simulink library "VehicleSimulation"  (R2014a)
settings: Solver=ode45  SolverMode=SingleTasking  StartTime=0.0  StopTime=10.0  RelTol=1e-3
undefined symbols (not defined in the file): bs, eff, fs, gpsins, gr, Js, kM, ljt, lma, param, rjt, rma, sglu, sr
libraries: simulink x2, VehicleSimulation x1
(part 1 of 2)
settings Model: Creator=Administrator  LastModifiedBy=cbeal

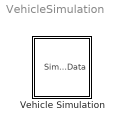
== system VehicleSimulation ==
  Vehicle Simulation : Subsystem  StopFcn=|  mask{InitPosE=9362.6, InitPosN=-418.6, InitYawAngle=-81.2, CruiseEnableTime=1, AutoSteerEnable=on, FaultEnable=off, HWHALEnable=off, TwoWheelEnable=on, DiffDriveEnable=off}
      | DataDescription = datadesc;                          
      | DataDescriptionSimulation=datadescSimulation;        
      |                                                      
      | %DataDescriptionUser = %datadescDriftController      
      |                                                      
      | %DataDescriptionUser = %datadescDriftSpeedController;
      |                                                      
      | DataDescriptionUser = datadescDriftkeeping;          
      |                                                      
      | %DataDescriptionUser = %datadescDriftControllerSDSC; 
      |                                                      
      | names;
      mask prompts: InitPosE "Initial East Position"; InitPosN "Initial North Position"; InitYawAngle "Initial Yaw Angle (deg)"; CruiseEnableTime "Cruise Control Enable Time (s)"; AutoSteerEnable "Enable Auto Steer"; FaultEnable "Enable Faults"; HWHALEnable "Enable HAL HW"; TwoWheelEnable "Use Two Wheel Model"; DiffDriveEnable "Use Differential Drive"
      mask help: This block provides a simulated hardware model.
      mask init:
      | InitModel;
      | p1_params;
      | ssest_params;
      | sim_params;
      | 
      | % TwoWheelSwitch_DriftControl = [gcs '/User Controllers' '/Drift and Speed Controller' '/Drift Controller Subsystem' '/Use Two Wheel Model'];
      | % TwoWheelSwitch_DriftControl = [gcs '/User Controllers' '/Simplified Drift Control' '/Drift Controller Subsystem' '/Use Two Wheel Model'];
      | % TwoWheelSwitch_DriftControl = [gcs '/User Controllers' '/Drift Control Block' '/Drift Controller Subsystem' '/Use Two Wheel Model'];
      | TwoWheelSwitch_DriftControl = [gcs '/User Controllers' '/Driftkeeping' '/Driftkeeping Subsystem' '/Use Two Wheel Model'];
      | TwoWheelSwitch_Sim = [gcs '/Vehicle Simulation' '/Vehicle Model' '/Use Two Wheel Model'];
      | DifferentialSwitch_Sim = [gcs '/Vehicle Simulation' '/Vehicle Model' '/Use Differential Drive'];
      | hwhal = [gcs '/Vehicle Simulation' '/Driver' '/Handwheel System' '/Enable HALHW'];
      | 
      | % default is turn off hwhal, two wheel model
      | set_param(hwhal, 'value', '0');
      | set_param(TwoWheelSwitch_DriftControl, 'value', '0');
      | set_param(TwoWheelSwitch_Sim, 'value', '0');
      | set_param(DifferentialSwitch_Sim, 'value', '0');
      | 
      | if (HWHALEnable == 1)
      |     set_param(hwhal, 'value', '1');
      | end
      | 
      | if (TwoWheelEnable == 1)
      |     set_param(TwoWheelSwitch_DriftControl, 'value', '1');
      |     set_param(TwoWheelSwitch_Sim, 'value', '1');
      | end
      | 
      | if (DiffDriveEnable == 1)
      |     set_param(DifferentialSwitch_Sim, 'value', '1');
      | end
      mask Display: disp('Sim');

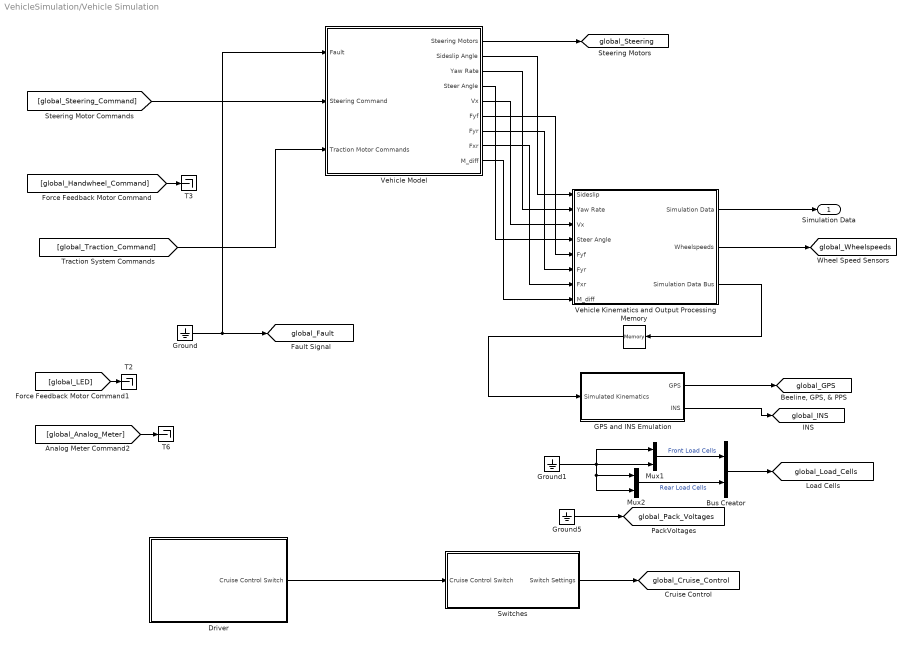
== system VehicleSimulation/Vehicle Simulation ==
  Bus Creator : BusCreator  Inputs=2
  Driver : Subsystem
  GPS and INS Emulation : Subsystem
  Ground : Ground
  Ground1 : Ground
  Ground5 : Ground
  Memory : Memory
  Mux1 : Mux  Inputs=2
  Mux2 : Mux  Inputs=2
  Switches : Subsystem
  T2 : Terminator
  T3 : Terminator
  T6 : Terminator
  Vehicle Kinematics and Output Processing : Subsystem
  Vehicle Model : Subsystem
  Simulation Data : Outport
  tag scope: global_Cruise_Control=global, global_Fault=global, global_GPS=global, global_INS=global, global_Load_Cells=global, global_Pack_Voltages=global, global_Steering=global, global_Wheelspeeds=global
  wires:
  Memory/1 -> GPS and INS Emulation/1(Simulated Kinematics)
  Vehicle Kinematics and Output Processing/3(Simulation Data Bus) -> Memory/1
  Vehicle Model/9(M_diff) -> Vehicle Kinematics and Output Processing/8(M_diff)
  Ground1/1 -> Mux2/2, Mux2/1, Mux1/2, Mux1/1
  GPS and INS Emulation/2(INS) -> [global_INS]
  GPS and INS Emulation/1(GPS) -> [global_GPS]
  Mux2/1 -> Bus Creator/2  "Rear Load Cells"
  Mux1/1 -> Bus Creator/1  "Front Load Cells"
  Driver/1(Cruise Control Switch) -> Switches/1(Cruise Control Switch)
  Vehicle Model/2(Sideslip Angle) -> Vehicle Kinematics and Output Processing/1(Sideslip)
  Vehicle Model/3(Yaw Rate) -> Vehicle Kinematics and Output Processing/2(Yaw Rate)
  Vehicle Model/1(Steering Motors) -> [global_Steering]
  Ground/1 -> Vehicle Model/1(Fault), [global_Fault]
  [global_Handwheel_Command] -> T3/1
  [global_LED] -> T2/1
  [global_Analog_Meter] -> T6/1
  Bus Creator/1 -> [global_Load_Cells]
  Ground5/1 -> [global_Pack_Voltages]
  Vehicle Kinematics and Output Processing/1(Simulation Data) -> Simulation Data/1
  Switches/1(Switch Settings) -> [global_Cruise_Control]
  [global_Steering_Command] -> Vehicle Model/2(Steering Command)
  Vehicle Model/4(Steer Angle) -> Vehicle Kinematics and Output Processing/4(Steer Angle)
  [global_Traction_Command] -> Vehicle Model/3(Traction Motor Commands)
  Vehicle Model/5(Vx) -> Vehicle Kinematics and Output Processing/3(Vx)
  Vehicle Model/6(Fyf) -> Vehicle Kinematics and Output Processing/5(Fyf)
  Vehicle Model/7(Fyr) -> Vehicle Kinematics and Output Processing/6(Fyr)
  Vehicle Model/8(Fxr) -> Vehicle Kinematics and Output Processing/7(Fxr)
  Vehicle Kinematics and Output Processing/2(Wheelspeeds) -> [global_Wheelspeeds]

== system VehicleSimulation/Vehicle Simulation/Driver ==
  Ground6 : Ground
  Handwheel System : Subsystem
  Pedal Voltage : Constant  Value=1.95
  Step : Step  Time=CruiseEnableTime  SampleTime=0
  Step1 : Step  Time=CruiseEnableTime+0.1  After=-1  SampleTime=0
  Sum : Sum  Inputs=+|+
  Cruise Control Switch : Outport
  tag scope: global_Go_Pedal=global, global_Handwheel=global, global_Prerecorded_Steering_Command=global
  wires:
  Step1/1 -> Sum/2
  Step/1 -> Sum/1
  Sum/1 -> Cruise Control Switch/1
  Ground6/1 -> [global_Prerecorded_Steering_Command]
  Pedal Voltage/1 -> [global_Go_Pedal]
  Handwheel System/1(Handwheel Signals) -> [global_Handwheel]

== system VehicleSimulation/Vehicle Simulation/GPS and INS Emulation ==
  Simulated Kinematics : Inport
  Bus Selector : BusSelector  OutputSignals=Yaw Rate,Heading,ax,ay,Vx,Vy,Pos E,Pos N
  Emulated INS : Subsystem
  GPS Emulation : Subsystem
  Radians to Degrees : Gain  Gain=180/pi
  Shift to Sensor/GPS Positions : Subsystem
  GPS : Outport
  INS : Outport  Port=2
  wires:
  Emulated INS/1(INS) -> INS/1
  GPS Emulation/1(Emulated GPS) -> GPS/1
  Shift to Sensor/GPS Positions/1(axINS) -> Emulated INS/2(axINS)
  Bus Selector/2 -> Radians to Degrees/1  "<Heading>"
  Radians to Degrees/1 -> GPS Emulation/1(Heading Angle)
  Bus Selector/4 -> Emulated INS/3(ay)  "<ay>"
  Bus Selector/8 -> GPS Emulation/5(Pos N)  "<Pos N>"
  Shift to Sensor/GPS Positions/2(VyGPS) -> GPS Emulation/3(VyGPS)
  Bus Selector/7 -> GPS Emulation/4(Pos E)  "<Pos E>"
  Bus Selector/6 -> Shift to Sensor/GPS Positions/3(Vy)  "<Vy>"
  Bus Selector/5 -> GPS Emulation/2(Vx)  "<Vx>"
  Bus Selector/3 -> Shift to Sensor/GPS Positions/2(ax)  "<ax>"
  Bus Selector/1 -> Emulated INS/1(Yaw Rate), Shift to Sensor/GPS Positions/1(Yaw Rate)  "<Yaw Rate>"
  Simulated Kinematics/1 -> Bus Selector/1

== system VehicleSimulation/Vehicle Simulation/Switches ==
  Cruise Control Switch : Inport
  Auto-Steer Switch : Constant  Value=AutoSteerEnable
  Brakes Disabled : Constant  Value=0
  Fault Switch : Constant  Value=FaultEnable
  Mux : Mux
  Switch Settings : Outport
  wires:
  Brakes Disabled/1 -> Mux/4  "Brake Pedal Signal"
  Auto-Steer Switch/1 -> Mux/2  "Auto-Steer Switch"
  Cruise Control Switch/1 -> Mux/3  "Cruise Control Switch"
  Fault Switch/1 -> Mux/1  "Fault Switch"
  Mux/1 -> Switch Settings/1

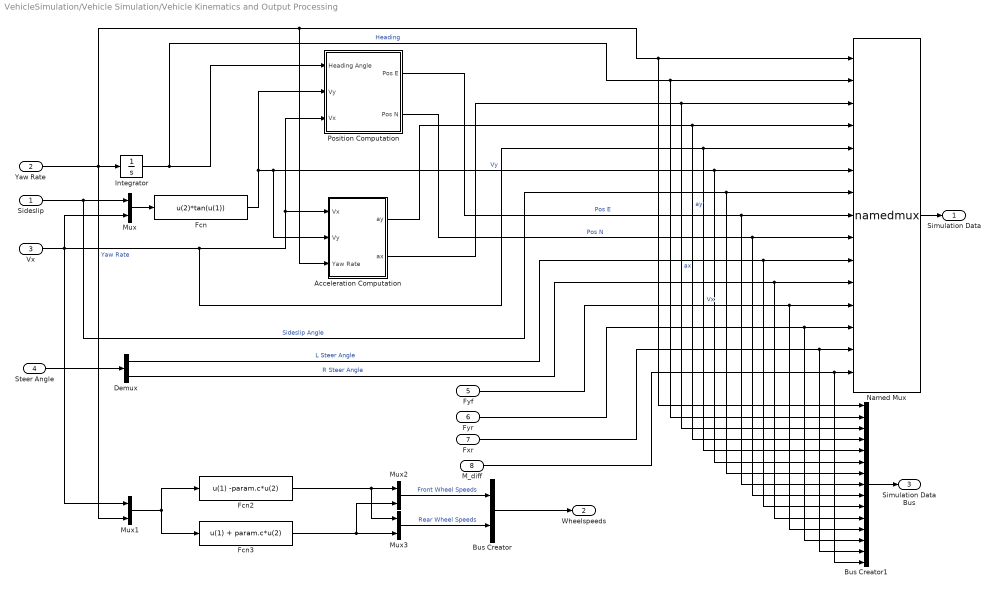
== system VehicleSimulation/Vehicle Simulation/Vehicle Kinematics and Output Processing ==
  Sideslip : Inport
  Yaw Rate : Inport  Port=2
  Vx : Inport  Port=3
  Steer Angle : Inport  Port=4
  Fyf : Inport  Port=5
  Fyr : Inport  Port=6
  Fxr : Inport  Port=7
  M_diff : Inport  Port=8
  Acceleration Computation : Subsystem
  Bus Creator : BusCreator  Inputs=2
  Bus Creator1 : BusCreator  Inputs=15
  Demux : Demux  Outputs=2
  Fcn : Fcn  Expr=u(2)*tan(u(1))
  Fcn2 : Fcn  Expr=u(1) -param.c*u(2)
  Fcn3 : Fcn  Expr=u(1) + param.c*u(2)
  Integrator : Integrator  InitialCondition=InitYawAngle*(pi/180)
  Mux{,1..3} (4 alike) : Mux  Inputs=2
  Named Mux : S-Function  FunctionName=namedmux  Parameters=inputcount,inputsizes  EnableBusSupport=off  mask{fname=datadescSimulation}
      mask prompts: fname "Data description function name"
      mask help:
      | Combines input signals into a single output vector, according to a structure that provides the names and sizes of each signal.
      |
      | The parameter below should be set to the name of a function which returns a 1xN structure array, where N is the number of input signals.  The structure should contain fields "size" which specifies the width of the input signal, and "name" which specifies its name.
      mask init:
      | desc=eval(fname);
      | %if(class(desc)~='cell')
      | %	error('Incorrect description');
      | %end
      | inputcount=length(desc);
      | if((inputcount<1)|(inputcount>50))
      | 	error('Inappropriate number of inputs.');
      | end
      | 
      | inputsizes=[desc.size];
      | 
      | x=min(inputcount*ones(1,50),1:50);
      mask Display:
      | port_label('input',x(1),desc(x(1)).name);
      | port_label('input',x(2),desc(x(2)).name);
      | port_label('input',x(3),desc(x(3)).name);
      | port_label('input',x(4),desc(x(4)).name);
      | port_label('input',x(5),desc(x(5)).name);
      | port_label('input',x(6),desc(x(6)).name);
      | port_label('input',x(7),desc(x(7)).name);
      | port_label('input',x(8),desc(x(8)).name);
      | port_label('input',x(9),desc(x(9)).name);
      | port_label('input',x(10),desc(x(10)).name);
      | port_label('input',x(11),desc(x(11)).name);
      | port_label('input',x(12),desc(x(12)).name);
      | port_label('input',x(13),desc(x(13)).name);
      | port_label('input',x(14),desc(x(14)).name);
      | port_label('input',x(15),desc(x(15)).name);
      | port_label('input',x(16),desc(x(16)).name);
      | port_label('input',x(17),desc(x(17)).name);
      | port_label('input',x(18),desc(x(18)).name);
      | port_label('input',x(19),desc(x(19)).name);
      | port_label('input',x(20),desc(x(20)).name);
      | port_label('input',x(21),desc(x(21)).name);
      | port_label('input',x(22),desc(x(22)).name);
      | port_label('input',x(23),desc(x(23)).name);
      | port_label('input',x(24),desc(x(24)).name);
      | port_label('input',x(25),desc(x(25)).name);
      | port_label('input',x(26),desc(x(26)).name);
      | port_label('input',x(27),desc(x(27)).name);
      | port_label('input',x(28),desc(x(28)).name);
      | port_label('input',x(29),desc(x(29)).name);
      | port_label('input',x(30),desc(x(30)).name);
  Position Computation : Subsystem
  Simulation Data : Outport
  Wheelspeeds : Outport  Port=2
  Simulation Data Bus : Outport  Port=3
  wires:
  M_diff/1 -> Bus Creator1/15, Named Mux/15
  Integrator/1 -> Position Computation/1(Heading Angle), Named Mux/2, Bus Creator1/2  "Heading"
  Fcn/1 -> Position Computation/2(Vy), Acceleration Computation/2(Vy), Named Mux/6, Bus Creator1/6  "Vy"
  Sideslip/1 -> Mux/1, Bus Creator1/7, Named Mux/7  "Sideslip Angle"
  Mux/1 -> Fcn/1
  Vx/1 -> Mux/2, Position Computation/3(Vx), Acceleration Computation/1(Vx), Named Mux/5, Bus Creator1/5, Mux1/1  "Vx"
  Yaw Rate/1 -> Acceleration Computation/3(Yaw Rate), Named Mux/1, Bus Creator1/1, Integrator/1, Mux1/2  "Yaw Rate"
  Position Computation/1(Pos E) -> Named Mux/8, Bus Creator1/8  "Pos E"
  Position Computation/2(Pos N) -> Named Mux/9, Bus Creator1/9  "Pos N"
  Named Mux/1 -> Simulation Data/1
  Steer Angle/1 -> Demux/1
  Demux/1 -> Named Mux/10, Bus Creator1/10  "L Steer Angle"
  Demux/2 -> Named Mux/11, Bus Creator1/11  "R Steer Angle"
  Acceleration Computation/1(ay) -> Named Mux/4, Bus Creator1/4  "ay"
  Acceleration Computation/2(ax) -> Named Mux/3, Bus Creator1/3  "ax"
  Fyf/1 -> Named Mux/12, Bus Creator1/12
  Fyr/1 -> Named Mux/13, Bus Creator1/13
  Fxr/1 -> Named Mux/14, Bus Creator1/14
  Mux1/1 -> Fcn2/1, Fcn3/1
  Fcn2/1 -> Mux2/1, Mux3/1
  Fcn3/1 -> Mux3/2, Mux2/2
  Mux2/1 -> Bus Creator/1  "Front Wheel Speeds"
  Mux3/1 -> Bus Creator/2  "Rear Wheel Speeds"
  Bus Creator/1 -> Wheelspeeds/1
  Bus Creator1/1 -> Simulation Data Bus/1

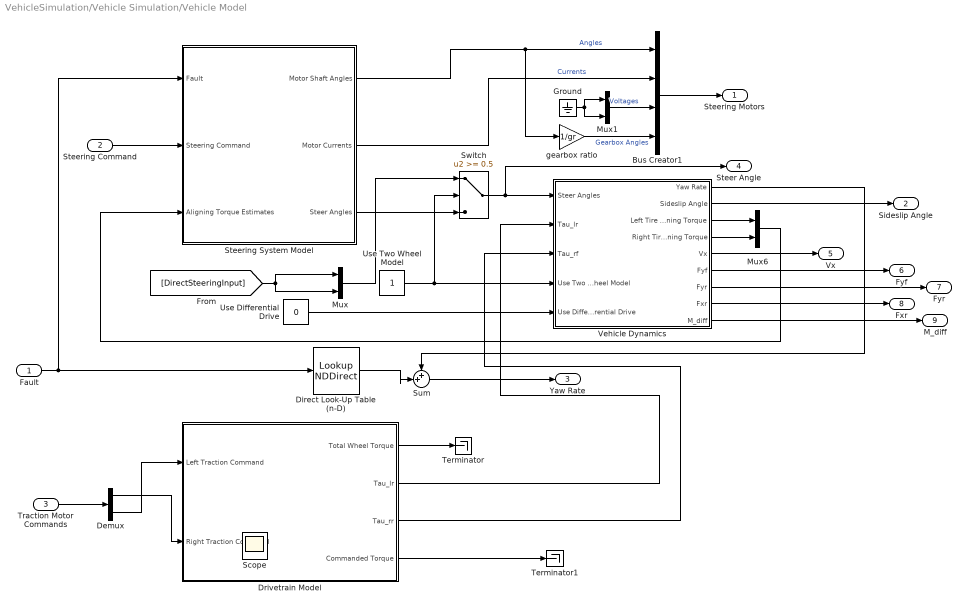
== system VehicleSimulation/Vehicle Simulation/Vehicle Model ==
  Fault : Inport
  Steering Command : Inport  Port=2
  Traction Motor Commands : Inport  Port=3
  Bus Creator1 : BusCreator
  Demux : Demux  Outputs=2
  Direct Look-Up Table (n-D) : LookupNDDirect  NumberOfTableDimensions=1  Table=[0 0 0 0 0 .01]
  Drivetrain Model : Subsystem
  Ground : Ground
  Mux : Mux  Inputs=2
  Mux1 : Mux  Inputs=2
  Mux6 : Mux  Inputs=2
  Scope : Scope
  Steering System Model : Subsystem
  Sum : Sum  Inputs=++|
  Switch : Switch  Threshold=0.5
  Terminator : Terminator
  Terminator1 : Terminator
  Use Differential Drive : Constant  Value=0
  Use Two Wheel Model : Constant
  Vehicle Dynamics : Subsystem
  gearbox ratio : Gain  Gain=1/gr  SaturateOnIntegerOverflow=on  OutDataTypeStr=Inherit: Same as input  ParamDataTypeStr=Inherit: Same as input
  Steering Motors : Outport
  Sideslip Angle : Outport  Port=2
  Yaw Rate : Outport  Port=3
  Steer Angle : Outport  Port=4
  Vx : Outport  Port=5
  Fyf : Outport  Port=6
  Fyr : Outport  Port=7
  Fxr : Outport  Port=8
  M_diff : Outport  Port=9
  wires:
  Drivetrain Model/3(Tau_rr) -> Vehicle Dynamics/3(Tau_rf)
  Drivetrain Model/2(Tau_lr) -> Vehicle Dynamics/2(Tau_lr)
  Vehicle Dynamics/9(M_diff) -> M_diff/1
  Traction Motor Commands/1 -> Demux/1
  Mux/1 -> Switch/1
  Steering System Model/3(Steer Angles) -> Switch/3
  Switch/1 -> Steer Angle/1, Vehicle Dynamics/1(Steer Angles)
  [DirectSteeringInput] -> Mux/2, Mux/1
  Vehicle Dynamics/2(Sideslip Angle) -> Sideslip Angle/1
  Sum/1 -> Yaw Rate/1
  Vehicle Dynamics/4(Right Tire Aligning Torque) -> Mux6/2
  Vehicle Dynamics/3(Left Tire Aligning Torque) -> Mux6/1
  Bus Creator1/1 -> Steering Motors/1
  Steering System Model/1(Motor Shaft Angles) -> Bus Creator1/1, gearbox ratio/1  "Angles"
  gearbox ratio/1 -> Bus Creator1/4  "Gearbox Angles"
  Steering System Model/2(Motor Currents) -> Bus Creator1/2  "Currents"
  Mux1/1 -> Bus Creator1/3  "Voltages"
  Direct Look-Up Table (n-D)/1 -> Sum/2
  Vehicle Dynamics/1(Yaw Rate) -> Sum/1
  Fault/1 -> Steering System Model/1(Fault), Direct Look-Up Table (n-D)/1
  Steering Command/1 -> Steering System Model/2(Steering Command)
  Mux6/1 -> Steering System Model/3(Aligning Torque Estimates)
  Vehicle Dynamics/5(Vx) -> Vx/1
  Drivetrain Model/1(Total Wheel Torque) -> Terminator/1
  Drivetrain Model/4(Commanded Torque) -> Terminator1/1
  Vehicle Dynamics/6(Fyf) -> Fyf/1
  Vehicle Dynamics/7(Fyr) -> Fyr/1
  Vehicle Dynamics/8(Fxr) -> Fxr/1
  Ground/1 -> Mux1/1, Mux1/2
  Use Two Wheel Model/1 -> Vehicle Dynamics/4(Use Two Wheel Model), Switch/2
  Use Differential Drive/1 -> Vehicle Dynamics/5(Use Differential Drive)
  Demux/2 -> Drivetrain Model/1(Left Traction Command)
  Demux/1 -> Drivetrain Model/2(Right Traction Command)

== system VehicleSimulation/Vehicle Simulation/Driver/Handwheel System ==
  Bus Creator3 : BusCreator  Inputs=3
  Enable HALHW : Constant  Value=0
  Ground : Ground
  Ground1 : Ground
  HAL-9000 : Subsystem  mask{enabled=on, maneuver=Step, amplitude=10, delay=10, duration=15, startfreq=.7, endfreq=.7}
      mask prompts: enabled "Enable HAL-9000 Automated Steering Maneuver System"; maneuver "Steering manuever"; amplitude "Amplitude (deg)"; delay "Delay (sec)"; duration "Duration (sec)"; startfreq "Initial frequency (Hz)"; endfreq "Final frequency (Hz)"
      mask init:
      | p1_params;
      | SteeringController;
      | 
      | switch(maneuver)
      | 	case 'Step'
      | 		maneuver=1;
      | 	case 'Ramp'
      | 		maneuver=2;
      | 	case 'Chirp'
      | 		maneuver=3;
      | 	case 'Double-step'
      | 		maneuver=4;
      | 	case 'Double chirp'
      | 		maneuver=5;
      | end
      | switch(enabled)
      | 	case 'on'
      | 		enabled=1;
      | 	case 'off'
      | 		enabled=0;
      | end
      mask Callback enabled:
      | if(strcmp(get_param(gcb,'enabled'),'off'))
      | 	set_param(gcb,'MaskEnables',{'on','off','off','off','off','off','off'});
      | else
      | 	set_param(gcb,'MaskEnables',{'on','on','on','on','on','on','on'});
      | end
      mask TypeOptions maneuver: Step | Ramp | Chirp | Double step | Double chirp
      mask Callback maneuver:
      | switch(get_param(gcb,'maneuver'))
      | 	case 'Step'
      | 		set_param(gcb,'MaskVisibilities',{'on','on','on','on','off','off','off'});
      | 	case 'Double step'
      | 		set_param(gcb,'MaskVisibilities',{'on','on','on','on','on','off','off'});
      | 	case 'Ramp'
      | 		set_param(gcb,'MaskVisibilities',{'on','on','on','on','on','off','off'});
      | 	case 'Chirp'
      | 		set_param(gcb,'MaskVisibilities',{'on','on','on','on','on','on','on'});
      | 	case 'Double chirp'
      | 		set_param(gcb,'MaskVisibilities',{'on','on','on','on','on','on','on'});
      | end
  Handwheel Signals : Outport
  wires:
  Enable HALHW/1 -> HAL-9000/1(Trigger)
  HAL-9000/1(Offset) -> Bus Creator3/1  "Primary"
  Ground/1 -> Bus Creator3/2  "First Backup"
  Bus Creator3/1 -> Handwheel Signals/1
  Ground1/1 -> Bus Creator3/3  "Second Backup"

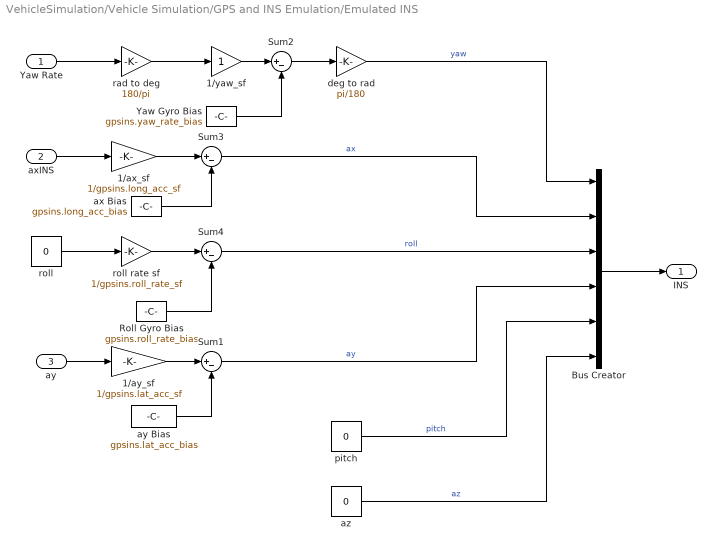
== system VehicleSimulation/Vehicle Simulation/GPS and INS Emulation/Emulated INS ==
  Yaw Rate : Inport
  axINS : Inport  Port=2
  ay : Inport  Port=3
  1/ax_sf : Gain  Gain=1/gpsins.long_acc_sf  SaturateOnIntegerOverflow=on  OutDataTypeStr=Inherit: Same as input  ParamDataTypeStr=Inherit: Same as input
  1/ay_sf : Gain  Gain=1/gpsins.lat_acc_sf  SaturateOnIntegerOverflow=on  OutDataTypeStr=Inherit: Same as input  ParamDataTypeStr=Inherit: Same as input
  1/yaw_sf : Gain
  Bus Creator : BusCreator  Inputs=6
  Roll Gyro Bias : Constant  Value=gpsins.roll_rate_bias
  Sum{1..4} (4 alike) : Sum  Inputs=|+-  SaturateOnIntegerOverflow=on  InputSameDT=on  OutDataTypeStr=Inherit: Same as first input
  Yaw Gyro Bias : Constant  Value=gpsins.yaw_rate_bias
  ax Bias : Constant  Value=gpsins.long_acc_bias
  ay Bias : Constant  Value=gpsins.lat_acc_bias
  az : Constant  Value=0
  deg to rad : Gain  Gain=pi/180
  pitch : Constant  Value=0
  rad to deg : Gain  Gain=180/pi
  roll : Constant  Value=0
  roll rate sf : Gain  Gain=1/gpsins.roll_rate_sf  SaturateOnIntegerOverflow=on  OutDataTypeStr=Inherit: Same as input  ParamDataTypeStr=Inherit: Same as input
  INS : Outport
  wires:
  Bus Creator/1 -> INS/1
  az/1 -> Bus Creator/6  "az"
  pitch/1 -> Bus Creator/5  "pitch"
  Sum4/1 -> Bus Creator/3  "roll"
  Roll Gyro Bias/1 -> Sum4/2
  roll rate sf/1 -> Sum4/1
  roll/1 -> roll rate sf/1
  Sum1/1 -> Bus Creator/4  "ay"
  Sum3/1 -> Bus Creator/2  "ax"
  deg to rad/1 -> Bus Creator/1  "yaw"
  ax Bias/1 -> Sum3/2
  1/ax_sf/1 -> Sum3/1
  axINS/1 -> 1/ax_sf/1
  ay Bias/1 -> Sum1/2
  1/ay_sf/1 -> Sum1/1
  ay/1 -> 1/ay_sf/1
  Sum2/1 -> deg to rad/1
  Yaw Gyro Bias/1 -> Sum2/2
  1/yaw_sf/1 -> Sum2/1
  rad to deg/1 -> 1/yaw_sf/1
  Yaw Rate/1 -> rad to deg/1

== system VehicleSimulation/Vehicle Simulation/GPS and INS Emulation/GPS Emulation ==
  Heading Angle : Inport
  Vx : Inport  Port=2
  VyGPS : Inport  Port=3
  Pos E : Inport  Port=4
  Pos N : Inport  Port=5
  Beeline Emulation : Subsystem
  Bus Creator : BusCreator  Inputs=5
  Clock : Clock
  OEM4 Emulation : Subsystem
  Pulse Generator : DiscretePulseGenerator  PulseType=Time based  Amplitude=4.1  Period=1  PulseWidth=50
  Sum : Sum  Inputs=|++
  UTC Offset : Constant  Value=250000
  Emulated GPS : Outport
  wires:
  OEM4 Emulation/3(OEM4 Other) -> Bus Creator/5  "OEM4 Other"
  OEM4 Emulation/1(OEM4 Position) -> Bus Creator/4  "OEM4 Position"
  Bus Creator/1 -> Emulated GPS/1
  Pulse Generator/1 -> Bus Creator/3  "PPS"
  OEM4 Emulation/2(OEM4 Velocity) -> Bus Creator/2  "OEM4 Velocity"
  Beeline Emulation/1(Beeline) -> Bus Creator/1  "Beeline"
  Pos N/1 -> OEM4 Emulation/5(Pos N)
  Pos E/1 -> OEM4 Emulation/4(Pos E)
  Heading Angle/1 -> Beeline Emulation/1("Heading Angle "), OEM4 Emulation/3(Heading Angle)
  VyGPS/1 -> Beeline Emulation/3(VyGPS), OEM4 Emulation/2(VyGPS)
  Vx/1 -> Beeline Emulation/2(Vx), OEM4 Emulation/1(Vx)
  Sum/1 -> OEM4 Emulation/6(UTC), Beeline Emulation/4(UTC)
  Clock/1 -> Sum/2
  UTC Offset/1 -> Sum/1

== system VehicleSimulation/Vehicle Simulation/GPS and INS Emulation/Shift to Sensor//GPS Positions ==
  Yaw Rate : Inport
  ax : Inport  Port=2
  Vy : Inport  Port=3
  "CG to INS Cube " : Fcn  Expr=u[2] + u[1]^2*gpsins.dist_sensor
  CG to INS Cube 1 : Fcn  Expr=u[2] -u[1]*gpsins.dist_sensor
  INS Cube to GPS Antenna : Fcn  Expr=u[2] + u[1]*gpsins.l_gps_ant
  Mux : Mux  Inputs=2
  Mux1 : Mux  Inputs=2
  Mux2 : Mux  Inputs=2
  axINS : Outport
  VyGPS : Outport  Port=2
  wires:
  "CG to INS Cube "/1 -> axINS/1
  INS Cube to GPS Antenna/1 -> VyGPS/1
  Vy/1 -> Mux1/2
  ax/1 -> Mux/2
  CG to INS Cube 1/1 -> Mux2/2
  Mux2/1 -> INS Cube to GPS Antenna/1
  Mux1/1 -> CG to INS Cube 1/1
  Mux/1 -> "CG to INS Cube "/1
  Yaw Rate/1 -> Mux2/1, Mux/1, Mux1/1

== system VehicleSimulation/Vehicle Simulation/Vehicle Kinematics and Output Processing/Acceleration Computation ==
  Vx : Inport
  Vy : Inport  Port=2
  Yaw Rate : Inport  Port=3
  Derivative : Derivative
  Derivative1 : Derivative
  Fcn1 : Fcn  Expr=u[1] + u[2]*u[3]
  Fcn2 : Fcn  Expr=u[1] - u[2]*u[3]
  Mux : Mux  Inputs=3
  Mux1 : Mux  Inputs=3
  ay : Outport
  ax : Outport  Port=2
  wires:
  Vx/1 -> Mux/3, Derivative/1
  Fcn1/1 -> ay/1
  Mux/1 -> Fcn1/1
  Fcn2/1 -> ax/1
  Mux1/1 -> Fcn2/1
  Derivative1/1 -> Mux/1
  Yaw Rate/1 -> Mux/2, Mux1/2
  Derivative/1 -> Mux1/1
  Vy/1 -> Derivative1/1, Mux1/3

== system VehicleSimulation/Vehicle Simulation/Vehicle Kinematics and Output Processing/Position Computation ==
  Heading Angle : Inport
  Vy : Inport  Port=2
  Vx : Inport  Port=3
  Compute Velocity East : Fcn  Expr=-u(3)*sin(u(1))-u(2)*cos(u(1))
  Computer Velocity North : Fcn  Expr=u(3)*cos(u(1))-u(2)*sin(u(1))
  Integrator : Integrator  InitialCondition=InitPosE
  Integrator1 : Integrator  InitialCondition=InitPosN
  Mux : Mux  Inputs=3
  Pos E : Outport
  Pos N : Outport  Port=2
  wires:
  Integrator1/1 -> Pos N/1
  Integrator/1 -> Pos E/1
  Mux/1 -> Computer Velocity North/1, Compute Velocity East/1
  Vx/1 -> Mux/3
  Vy/1 -> Mux/2
  Heading Angle/1 -> Mux/1
  Compute Velocity East/1 -> Integrator/1
  Computer Velocity North/1 -> Integrator1/1

== system VehicleSimulation/Vehicle Simulation/Vehicle Model/Drivetrain Model ==
  Left Traction Command : Inport
  Right Traction Command : Inport  Port=2
  Drivetrain Model : Subsystem  TreatAsAtomicUnit=on
  Lookup Table : Lookup  InputValues=[0.9,1.7,2.8]  Table=[-70.5,0,190.5]  LookUpMeth=Interpolation-Use End Values
  Lookup Table1 : Lookup  InputValues=[0.9,1.7,2.8]  Table=[-70.5,0,190.5]  LookUpMeth=Interpolation-Use End Values
  Saturation : Saturate  UpperLimit=2.8  LowerLimit=0.9
  Saturation1 : Saturate  UpperLimit=2.8  LowerLimit=0.9
  Total Wheel Torque : Outport
  Tau_lr : Outport  Port=2
  Tau_rr : Outport  Port=3
  Commanded Torque : Outport  Port=4
  wires:
  Lookup Table1/1 -> Drivetrain Model/2(Motor 2 Torque Request)
  Right Traction Command/1 -> Saturation1/1
  Saturation1/1 -> Lookup Table1/1
  Lookup Table/1 -> Drivetrain Model/1(Motor 1 Torque Request)
  Left Traction Command/1 -> Saturation/1
  Saturation/1 -> Lookup Table/1
  Drivetrain Model/1(Total Wheel Torque) -> Total Wheel Torque/1
  Drivetrain Model/2(Tau_lr) -> Tau_lr/1
  Drivetrain Model/3(Tau_rr) -> Tau_rr/1

== system VehicleSimulation/Vehicle Simulation/Vehicle Model/Steering System Model ==
  Fault : Inport
  Steering Command : Inport  Port=2
  Aligning Torque Estimates : Inport  Port=3
  Electrical Components and Motors : Subsystem
  Jacking Torques : Subsystem
      mask init:
      | % Generate the lookup tables
      | p1_params
      | nissan_steer_lookup_data
      mask Display: disp('.')
  Motor Shaft Angles to Steer Angles : Subsystem
      mask init:
      | % Generate the lookup tables
      | p1_params
      | nissan_steer_lookup_data
      mask Display: disp('.')
  Sum : Sum  Inputs=|++  SaturateOnIntegerOverflow=on
  Terminator : Terminator
  Motor Shaft Angles : Outport
  Motor Currents : Outport  Port=2
  Steer Angles : Outport  Port=3
  wires:
  Fault/1 -> Electrical Components and Motors/1(Fault)
  Motor Shaft Angles to Steer Angles/1(Steer Angles) -> Steer Angles/1
  Electrical Components and Motors/2(Motor Currents) -> Motor Currents/1
  Electrical Components and Motors/3(True Angles) -> Jacking Torques/1(Motor Shaft Angles), Motor Shaft Angles/1, Motor Shaft Angles to Steer Angles/1(Motor Shaft Angles)
  Steering Command/1 -> Electrical Components and Motors/2(Steering Command)
  Sum/1 -> Electrical Components and Motors/3(Torques)
  Electrical Components and Motors/1(Sensed Angles) -> Terminator/1
  Jacking Torques/1(Jacking Torques) -> Sum/2
  Aligning Torque Estimates/1 -> Sum/1

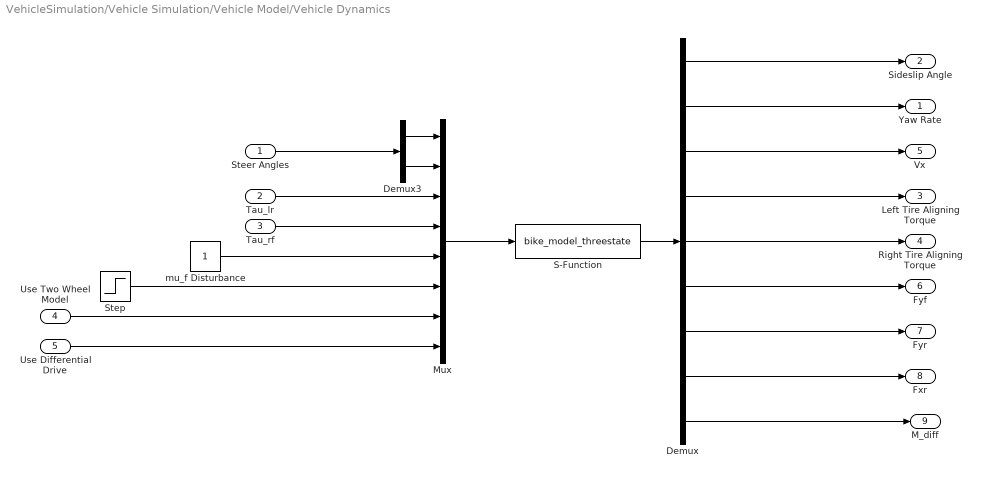
== system VehicleSimulation/Vehicle Simulation/Vehicle Model/Vehicle Dynamics ==
  Steer Angles : Inport
  Tau_lr : Inport  Port=2
  Tau_rf : Inport  Port=3
  Use Two Wheel Model : Inport  Port=4
  Use Differential Drive : Inport  Port=5
  Demux : Demux  Outputs=9
  Demux3 : Demux  Outputs=2
  Mux : Mux  Inputs=8
  S-Function : S-Function  FunctionName=bike_model_threestate  Parameters=param.fl.C, param.fr.C, param.rl.C, param.rr.C, param.m, param.Iz, param.a, param.b,param.c, tp,tm,simparam.mu_p_f,simparam.mu_s_f,simparam.mu_p_r,simparam.mu_s_r,param.rl.r  EnableBusSupport=off
  Step : Step  Time=35  Before=1  SampleTime=0
  mu_f Disturbance : Constant
  Yaw Rate : Outport
  Sideslip Angle : Outport  Port=2
  Left Tire Aligning Torque : Outport  Port=3
  Right Tire Aligning Torque : Outport  Port=4
  Vx : Outport  Port=5
  Fyf : Outport  Port=6
  Fyr : Outport  Port=7
  Fxr : Outport  Port=8
  M_diff : Outport  Port=9
  wires:
  Demux/9 -> M_diff/1
  Use Differential Drive/1 -> Mux/8
  Use Two Wheel Model/1 -> Mux/7
  Step/1 -> Mux/6
  mu_f Disturbance/1 -> Mux/5
  Demux/1 -> Sideslip Angle/1
  Demux/2 -> Yaw Rate/1
  Demux3/2 -> Mux/2
  Demux3/1 -> Mux/1
  S-Function/1 -> Demux/1
  Steer Angles/1 -> Demux3/1
  Tau_lr/1 -> Mux/3
  Tau_rf/1 -> Mux/4
  Demux/3 -> Vx/1
  Demux/4 -> Left Tire Aligning Torque/1
  Demux/5 -> Right Tire Aligning Torque/1
  Mux/1 -> S-Function/1
  Demux/6 -> Fyf/1
  Demux/7 -> Fyr/1
  Demux/8 -> Fxr/1

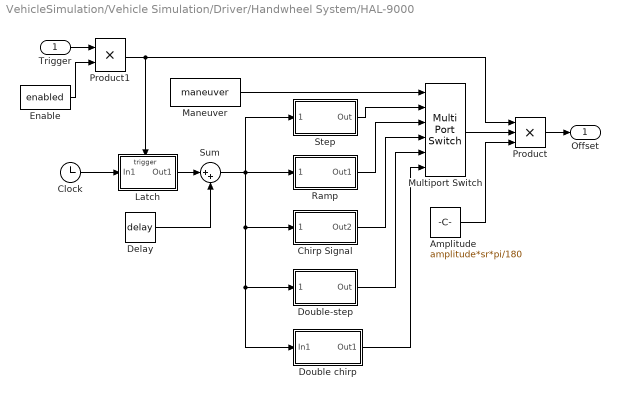
== system VehicleSimulation/Vehicle Simulation/Driver/Handwheel System/HAL-9000 ==
  Trigger : Inport
  Amplitude : Constant  Value=amplitude*sr*pi/180
  Chirp Signal : Subsystem  mask(chirp){f1=startfreq, T=duration, f2=endfreq, VectorParams1D=on}
      mask prompts: f1 "Initial frequency (Hz):"; T "Target time (secs):"; f2 "Frequency at target time (Hz):"; VectorParams1D "Interpret vectors parameters as 1-D"
      mask help: Output a linear chirp signal (sine wave whose frequency varies linearly with time).
      mask init:
      | blkName = gcb;
      | t=[0:.1:5];
      | set_param([blkName '/targetTime'], 'VectorParams1D', VectorParams1D);
      | set_param([blkName '/initialFreq'], 'VectorParams1D', VectorParams1D);
      | set_param([blkName '/deltaFreq'], 'VectorParams1D', VectorParams1D);
      mask Help: The chirp signal has linearly increasing frequency with time.  This block can be used for spectral analysis of nonlinear systems.
      mask Display: plot(t,sin(t.*t))
  Clock : Clock
  Delay : Constant  Value=delay
  Double chirp : Subsystem
  Double-step : Subsystem
      mask Display: plot([0 1 1 2 2 3 3 4 4 5],[0 0 1 1 0 0 -1 -1 0 0])
  Enable : Constant  Value=enabled
  Latch : Subsystem  TreatAsAtomicUnit=on
  Maneuver : Constant  Value=maneuver
  Multiport Switch : MultiPortSwitch  Inputs=5
  Product : Product  Inputs=3  SaturateOnIntegerOverflow=on  OutDataTypeStr=Inherit: Same as first input
  Product1 : Product  SaturateOnIntegerOverflow=on  OutDataTypeStr=Inherit: Same as first input
  Ramp : Subsystem
      mask Display: plot([0 3 7 10],[1 1 8 8])
  Step : Subsystem
      mask Display: plot([0 5 5 10],[1 1 8 8])
  Sum : Sum  Inputs=|++
  Offset : Outport
  wires:
  Double chirp/1(Out1) -> Multiport Switch/6
  Double-step/1(Out) -> Multiport Switch/5
  Enable/1 -> Product1/2
  Trigger/1 -> Product1/1
  Delay/1 -> Sum/2
  Latch/1(Out1) -> Sum/1
  Chirp Signal/1(Out2) -> Multiport Switch/4
  Ramp/1(Out1) -> Multiport Switch/3
  Sum/1 -> Double chirp/1(In1), Double-step/1(Start Time), Chirp Signal/1(Start Time), Ramp/1(Start Time), Step/1(Start Time)
  Maneuver/1 -> Multiport Switch/1
  Step/1(Out) -> Multiport Switch/2
  Amplitude/1 -> Product/3
  Multiport Switch/1 -> Product/2
  Product/1 -> Offset/1
  Product1/1 -> Latch/Trigger, Product/1
  Clock/1 -> Latch/1(In1)

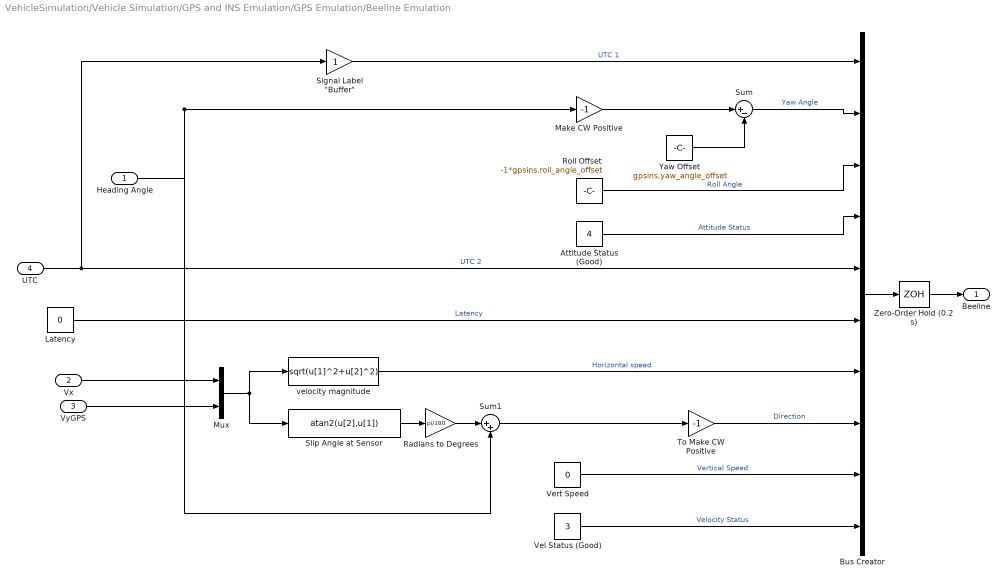
== system VehicleSimulation/Vehicle Simulation/GPS and INS Emulation/GPS Emulation/Beeline Emulation ==
  "Heading Angle " : Inport
  Vx : Inport  Port=2
  VyGPS : Inport  Port=3
  UTC : Inport  Port=4
  Attitude Status (Good) : Constant  Value=4
  Bus Creator : BusCreator  Inputs=10
  Latency : Constant  Value=0
  Make CW Positive : Gain  Gain=-1
  Mux : Mux  Inputs=2
  Radians to Degrees : Gain  Gain=pi/180
  Roll Offset : Constant  Value=-1*gpsins.roll_angle_offset
  "Signal Label \"Buffer\"" : Gain
  Slip Angle at Sensor : Fcn  Expr=atan2(u[2],u[1])
  Sum : Sum  Inputs=|+-
  Sum1 : Sum  Inputs=|++
  To Make CW Positive : Gain  Gain=-1
  Vel Status (Good) : Constant  Value=3
  Vert Speed : Constant  Value=0
  Yaw Offset : Constant  Value=gpsins.yaw_angle_offset
  "Zero-Order Hold (0.2 s) " : ZeroOrderHold  SampleTime=0.2
  velocity magnitude : Fcn  Expr=sqrt(u[1]^2+u[2]^2)
  Beeline : Outport
  wires:
  Sum1/1 -> To Make CW Positive/1
  Radians to Degrees/1 -> Sum1/1
  Slip Angle at Sensor/1 -> Radians to Degrees/1
  "Zero-Order Hold (0.2 s) "/1 -> Beeline/1
  Bus Creator/1 -> "Zero-Order Hold (0.2 s) "/1
  "Signal Label \"Buffer\""/1 -> Bus Creator/1  "UTC 1"
  Attitude Status (Good)/1 -> Bus Creator/4  "Attitude Status"
  Roll Offset/1 -> Bus Creator/3  "Roll Angle"
  Vel Status (Good)/1 -> Bus Creator/10  "Velocity Status"
  To Make CW Positive/1 -> Bus Creator/8  "Direction"
  Vert Speed/1 -> Bus Creator/9  "Vertical Speed"
  velocity magnitude/1 -> Bus Creator/7  "Horizontal speed"
  Latency/1 -> Bus Creator/6  "Latency"
  UTC/1 -> Bus Creator/5, "Signal Label \"Buffer\""/1  "UTC 2"
  Mux/1 -> velocity magnitude/1, Slip Angle at Sensor/1
  VyGPS/1 -> Mux/2
  Vx/1 -> Mux/1
  Sum/1 -> Bus Creator/2  "Yaw Angle"
  Yaw Offset/1 -> Sum/2
  Make CW Positive/1 -> Sum/1
  "Heading Angle "/1 -> Make CW Positive/1, Sum1/2

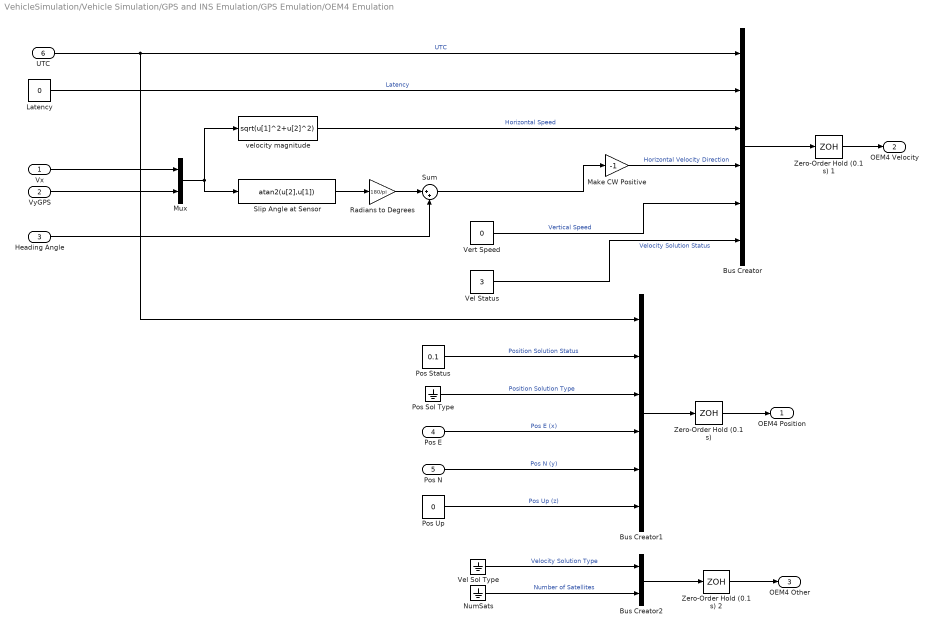
== system VehicleSimulation/Vehicle Simulation/GPS and INS Emulation/GPS Emulation/OEM4 Emulation ==
  Vx : Inport
  VyGPS : Inport  Port=2
  Heading Angle : Inport  Port=3
  Pos E : Inport  Port=4
  Pos N : Inport  Port=5
  UTC : Inport  Port=6
  " Make CW Positive" : Gain  Gain=-1
  Bus Creator : BusCreator  Inputs=6
  Bus Creator1 : BusCreator  Inputs=6
  Bus Creator2 : BusCreator  Inputs=2
  Latency : Constant  Value=0
  Mux : Mux  Inputs=2
  NumSats : Ground
  Pos Sol Type : Ground
  Pos Status : Constant  Value=0.1
  Pos Up : Constant  Value=0
  Radians to Degrees : Gain  Gain=180/pi
  Slip Angle at Sensor : Fcn  Expr=atan2(u[2],u[1])
  Sum : Sum  Inputs=|++
  Vel Sol Type : Ground
  Vel Status : Constant  Value=3
  Vert Speed : Constant  Value=0
  Zero-Order Hold (0.1 s) : ZeroOrderHold  SampleTime=0.1
  Zero-Order Hold (0.1 s) 1 : ZeroOrderHold  SampleTime=0.1
  Zero-Order Hold (0.1 s) 2 : ZeroOrderHold  SampleTime=0.1
  velocity magnitude : Fcn  Expr=sqrt(u[1]^2+u[2]^2)
  OEM4 Position : Outport
  OEM4 Velocity : Outport  Port=2
  OEM4 Other : Outport  Port=3
  wires:
  Sum/1 -> " Make CW Positive"/1
  Radians to Degrees/1 -> Sum/1
  Slip Angle at Sensor/1 -> Radians to Degrees/1
  Vel Status/1 -> Bus Creator/6  "Velocity Solution Status"
  Zero-Order Hold (0.1 s) 2/1 -> OEM4 Other/1
  Bus Creator2/1 -> Zero-Order Hold (0.1 s) 2/1
  Zero-Order Hold (0.1 s) 1/1 -> OEM4 Velocity/1
  Bus Creator/1 -> Zero-Order Hold (0.1 s) 1/1
  Zero-Order Hold (0.1 s)/1 -> OEM4 Position/1
  Bus Creator1/1 -> Zero-Order Hold (0.1 s)/1
  NumSats/1 -> Bus Creator2/2  "Number of Satellites"
  Vel Sol Type/1 -> Bus Creator2/1  "Velocity Solution Type"
  Pos Up/1 -> Bus Creator1/6  "Pos Up (z)"
  Pos N/1 -> Bus Creator1/5  "Pos N (y)"
  Pos E/1 -> Bus Creator1/4  "Pos E (x)"
  Pos Sol Type/1 -> Bus Creator1/3  "Position Solution Type"
  Pos Status/1 -> Bus Creator1/2  "Position Solution Status"
  " Make CW Positive"/1 -> Bus Creator/4  "Horizontal Velocity Direction"
  Vert Speed/1 -> Bus Creator/5  "Vertical Speed"
  velocity magnitude/1 -> Bus Creator/3  "Horizontal Speed"
  Latency/1 -> Bus Creator/2  "Latency"
  UTC/1 -> Bus Creator/1, Bus Creator1/1  "UTC"
  Heading Angle/1 -> Sum/2
  Mux/1 -> velocity magnitude/1, Slip Angle at Sensor/1
  VyGPS/1 -> Mux/2
  Vx/1 -> Mux/1

== system VehicleSimulation/Vehicle Simulation/Vehicle Model/Drivetrain Model/Drivetrain Model ==
  Motor 1 Torque Request : Inport
  Motor 2 Torque Request : Inport  Port=2
  Gearbox 1 : Subsystem  mask{ratio=5.5, efficiency=1}
      mask prompts: ratio "Gear Ratio"; efficiency "Transmission Efficiency"
  Gearbox 2 : VehicleSimulation/Vehicle Simulation/Vehicle Model/Drivetrain Model/Drivetrain Model/Gearbox 1  ratio=5.5  efficiency=1
  Sum2 : Sum
  Total Wheel Torque : Outport
  Tau_lr : Outport  Port=2
  Tau_rr : Outport  Port=3
  wires:
  Sum2/1 -> Total Wheel Torque/1
  Gearbox 1/1(Wheel Torque) -> Sum2/1, Tau_lr/1
  Gearbox 2/1 -> Sum2/2, Tau_rr/1
  Motor 1 Torque Request/1 -> Gearbox 1/1(Torque Request)
  Motor 2 Torque Request/1 -> Gearbox 2/1

== system VehicleSimulation/Vehicle Simulation/Vehicle Model/Steering System Model/Electrical Components and Motors ==
  Fault : Inport
  Steering Command : Inport  Port=2
  Torques : Inport  Port=3
  Amplifiers : Subsystem
      mask init:
      | amplifier_params
  Motors : Subsystem
  Sensed Angles : Outport
  Motor Currents : Outport  Port=2
  True Angles : Outport  Port=3
  wires:
  Amplifiers/1(Current Input) -> Motors/3(Current Input)
  Motors/3(Currents) -> Motor Currents/1
  Fault/1 -> Motors/1(Fault)
  Motors/2(Sensed Angles) -> Sensed Angles/1
  Steering Command/1 -> Amplifiers/1(Current Commands)
  Torques/1 -> Motors/2(Load Torques)
  Motors/1(Angles) -> True Angles/1

== system VehicleSimulation/Vehicle Simulation/Vehicle Model/Steering System Model/Jacking Torques ==
  Motor Shaft Angles : Inport
  Demux1 : Demux  Outputs=2
  Gain : Gain  Gain=1/gr  SaturateOnIntegerOverflow=on  OutDataTypeStr=Inherit: Same as input  ParamDataTypeStr=Inherit: Same as input
  Left-hand look-up table : Lookup  InputValues=lma  Table=ljt  SaturateOnIntegerOverflow=on
  Mux6 : Mux  Inputs=2
  Right-hand look-up table : Lookup  InputValues=rma  Table=rjt  SaturateOnIntegerOverflow=on
  Jacking Torques : Outport
  wires:
  Motor Shaft Angles/1 -> Gain/1
  Gain/1 -> Demux1/1
  Demux1/1 -> Left-hand look-up table/1
  Mux6/1 -> Jacking Torques/1
  Left-hand look-up table/1 -> Mux6/1
  Demux1/2 -> Right-hand look-up table/1
  Right-hand look-up table/1 -> Mux6/2

== system VehicleSimulation/Vehicle Simulation/Vehicle Model/Steering System Model/Motor Shaft Angles to Steer Angles ==
  Motor Shaft Angles : Inport
  Demux1 : Demux  Outputs=2
  Gain : Gain  Gain=1/gr  SaturateOnIntegerOverflow=on  OutDataTypeStr=Inherit: Same as input  ParamDataTypeStr=Inherit: Same as input
  Left-hand look-up table : Lookup  InputValues=sglu.fl.ma  Table=sglu.fl.sa  SaturateOnIntegerOverflow=on
  Mux6 : Mux  Inputs=2
  Right-hand look-up table : Lookup  InputValues=sglu.fr.ma  Table=sglu.fr.sa  SaturateOnIntegerOverflow=on
  Steer Angles : Outport
  wires:
  Right-hand look-up table/1 -> Mux6/2
  Demux1/2 -> Right-hand look-up table/1
  Left-hand look-up table/1 -> Mux6/1
  Mux6/1 -> Steer Angles/1
  Demux1/1 -> Left-hand look-up table/1
  Gain/1 -> Demux1/1
  Motor Shaft Angles/1 -> Gain/1

== system VehicleSimulation/Vehicle Simulation/Driver/Handwheel System/HAL-9000/Chirp Signal ==
  note: freqSlope = deltaFreq/targetTime;
      | instantaneousFreq(t) = freqSlope*t + initialFreq;
      | intantaneousPhase(t) = integral(instFreq) = ...
      |       0.5*freqSlope*t^2 + initialFreq*t;
      | outputSignal(t) = sin(instantaneousPhase(t));
  Start Time : Inport
  Clock1 : Clock
      settings: DisableCoverage=on
  Gain : Gain  DisableCoverage=on  Gain=0.5  OutDataTypeStr=Inherit: Same as input  ParamDataTypeStr=Inherit: Same as input
  Output : Trigonometry
  Product : Product  DisableCoverage=on  Inputs=*/  SaturateOnIntegerOverflow=on  InputSameDT=on  OutDataTypeStr=Inherit: Same as first input
  Product1 : Product  DisableCoverage=on  SaturateOnIntegerOverflow=on  InputSameDT=on  OutDataTypeStr=Inherit: Same as first input
  Product2 : Product  DisableCoverage=on  SaturateOnIntegerOverflow=on  InputSameDT=on  OutDataTypeStr=Inherit: Same as first input
  Saturation : Saturate  UpperLimit=duration  LowerLimit=0
  Sum : Sum  DisableCoverage=on  Inputs=|++  SaturateOnIntegerOverflow=on  InputSameDT=on  OutDataTypeStr=Inherit: Same as first input
  Sum1 : Sum  DisableCoverage=on  Inputs=-+|  SaturateOnIntegerOverflow=on  InputSameDT=on  OutDataTypeStr=Inherit: Same as first input
  deltaFreq : Constant  DisableCoverage=on  Value=2*pi*(f2-f1)
  initialFreq : Constant  DisableCoverage=on  Value=2*pi*f1
  targetTime : Constant  DisableCoverage=on  Value=T
  Out2 : Outport
  wires:
  Sum1/1 -> Saturation/1
  Clock1/1 -> Sum1/2
  Start Time/1 -> Sum1/1
  deltaFreq/1 -> Product/1
  targetTime/1 -> Product/2
  Product/1 -> Gain/1
  Gain/1 -> Product1/2
  Product1/1 -> Sum/1
  initialFreq/1 -> Sum/2
  Sum/1 -> Product2/2
  Product2/1 -> Output/1
  Output/1 -> Out2/1
  Saturation/1 -> Product1/1, Product2/1

== system VehicleSimulation/Vehicle Simulation/Driver/Handwheel System/HAL-9000/Double chirp ==
  In1 : Inport
  Chirp One : Subsystem  mask(chirp){f1=startfreq, T=duration/2, f2=endfreq, VectorParams1D=on}
      mask prompts: f1 "Initial frequency (Hz):"; T "Target time (secs):"; f2 "Frequency at target time (Hz):"; VectorParams1D "Interpret vectors parameters as 1-D"
      mask help: Output a linear chirp signal (sine wave whose frequency varies linearly with time).
      mask init: same as VehicleSimulation/Vehicle Simulation/Driver/Handwheel System/HAL-9000/Chirp Signal
      mask Help: The chirp signal has linearly increasing frequency with time.  This block can be used for spectral analysis of nonlinear systems.
      mask Display: plot(t,sin(t.*t))
  Chirp Two : Subsystem  mask(chirp){f1=startfreq, T=duration/2, f2=endfreq, VectorParams1D=on}
      mask prompts: f1 "Initial frequency (Hz):"; T "Target time (secs):"; f2 "Frequency at target time (Hz):"; VectorParams1D "Interpret vectors parameters as 1-D"
      mask help: Output a linear chirp signal (sine wave whose frequency varies linearly with time).
      mask init: same as VehicleSimulation/Vehicle Simulation/Driver/Handwheel System/HAL-9000/Chirp Signal
      mask Help: The chirp signal has linearly increasing frequency with time.  This block can be used for spectral analysis of nonlinear systems.
      mask Display: plot(t,sin(t.*t))
  Clock : Clock
  Relational Operator : RelationalOperator  Operator=<=  OutDataTypeStr=float('double')
  Sum : Sum  DisableCoverage=on  Inputs=++|  SaturateOnIntegerOverflow=on  InputSameDT=on  OutDataTypeStr=Inherit: Same as first input
  Switch : Switch  Threshold=.5
  initialFreq : Constant  DisableCoverage=on  Value=duration/2
  Out1 : Outport
  wires:
  Clock/1 -> Relational Operator/1
  Relational Operator/1 -> Switch/2
  initialFreq/1 -> Sum/2
  Sum/1 -> Relational Operator/2, Chirp Two/1(Start Time)
  In1/1 -> Sum/1, Chirp One/1(Start Time)
  Switch/1 -> Out1/1
  Chirp Two/1(Out2) -> Switch/3
  Chirp One/1(Out2) -> Switch/1

== system VehicleSimulation/Vehicle Simulation/Driver/Handwheel System/HAL-9000/Double-step ==
  Start Time : Inport
  Clock : Clock
  Data Type Conversion : DataTypeConversion  OutDataTypeStr=double
  Data Type Conversion1 : DataTypeConversion  OutDataTypeStr=double
  Left Pulse : simulink/Logic and Bit Operations/Interval Test  IntervalClosedRight=off  uplimit=duration  IntervalClosedLeft=on  lowlimit=0  OutDataTypeStr=boolean
  Right Pulse : simulink/Logic and Bit Operations/Interval Test  IntervalClosedRight=off  uplimit=3*duration  IntervalClosedLeft=on  lowlimit=2*duration  OutDataTypeStr=boolean
  Sum : Sum  Inputs=+|-
  Sum1 : Sum  Inputs=+|-
  Out : Outport
  wires:
  Data Type Conversion1/1 -> Sum1/2
  Data Type Conversion/1 -> Sum1/1
  Left Pulse/1 -> Data Type Conversion/1
  Right Pulse/1 -> Data Type Conversion1/1
  Sum1/1 -> Out/1
  Sum/1 -> Right Pulse/1, Left Pulse/1
  Clock/1 -> Sum/1
  Start Time/1 -> Sum/2

== system VehicleSimulation/Vehicle Simulation/Driver/Handwheel System/HAL-9000/Latch ==
  In1 : Inport
  Trigger : TriggerPort
  Out1 : Outport
  wires:
  In1/1 -> Out1/1

== system VehicleSimulation/Vehicle Simulation/Driver/Handwheel System/HAL-9000/Ramp ==
  Start Time : Inport
  Clock : Clock
      settings: DisableCoverage=on
  Saturation : Saturate  UpperLimit=1  LowerLimit=0
  Slope : Gain  Gain=1/duration
  Sum : Sum  DisableCoverage=on  Inputs=|+-  SaturateOnIntegerOverflow=on  InputSameDT=on  OutDataTypeStr=Inherit: Same as first input
  Out1 : Outport
  wires:
  Slope/1 -> Saturation/1
  Saturation/1 -> Out1/1
  Sum/1 -> Slope/1
  Start Time/1 -> Sum/2
  Clock/1 -> Sum/1

== system VehicleSimulation/Vehicle Simulation/Driver/Handwheel System/HAL-9000/Step ==
  Start Time : Inport
  Clock : Clock
  Relational Operator : RelationalOperator  OutDataTypeStr=float('double')
  Out : Outport
  wires:
  Start Time/1 -> Relational Operator/2
  Clock/1 -> Relational Operator/1
  Relational Operator/1 -> Out/1

== system VehicleSimulation/Vehicle Simulation/Vehicle Model/Drivetrain Model/Drivetrain Model/Gearbox 1 ==
  Torque Request : Inport
  Gear Ratio : Constant  Value=ratio
  Gearbox Efficiency : Constant  Value=efficiency
  Geared Torque : Product  RndMeth=Zero
  Inverter Input Power3 : Product  RndMeth=Zero
  Wheel Torque : Outport
  wires:
  Gear Ratio/1 -> Geared Torque/1
  Torque Request/1 -> Geared Torque/2
  Geared Torque/1 -> Inverter Input Power3/1
  Inverter Input Power3/1 -> Wheel Torque/1
  Gearbox Efficiency/1 -> Inverter Input Power3/2

== system VehicleSimulation/Vehicle Simulation/Vehicle Model/Steering System Model/Electrical Components and Motors/Amplifiers ==
  Current Commands : Inport
  Demux1 : Demux  Outputs=2
  Left Amplifier : Subsystem
  Mux : Mux  Inputs=2
  Right Amplifier : Subsystem
  Current Input : Outport
  wires:
  Mux/1 -> Current Input/1
  Right Amplifier/1(Current Input) -> Mux/2
  Left Amplifier/1(Current Input) -> Mux/1
  Demux1/2 -> Right Amplifier/1(Current Command1)
  Current Commands/1 -> Demux1/1
  Demux1/1 -> Left Amplifier/1(Current Command)

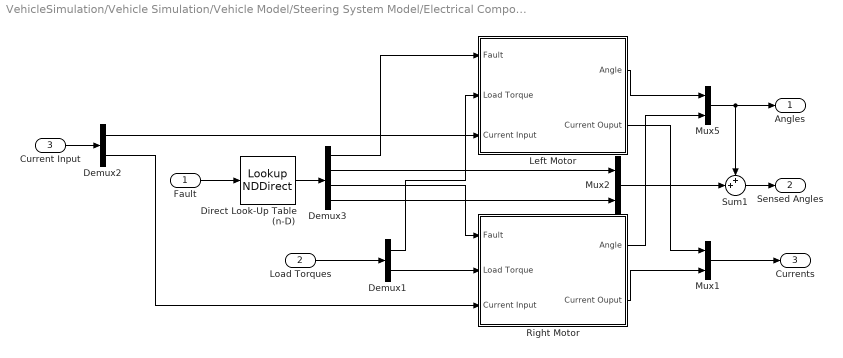
== system VehicleSimulation/Vehicle Simulation/Vehicle Model/Steering System Model/Electrical Components and Motors/Motors ==
  Fault : Inport
  Load Torques : Inport  Port=2
  Current Input : Inport  Port=3
  Demux1 : Demux  Outputs=2
  Demux2 : Demux  Outputs=2
  Demux3 : Demux
  Direct Look-Up Table (n-D) : LookupNDDirect  InputsSelectThisObjectFromTable=Column  Table=[0 1 0 0 0 0; 0 0 0 14 0 0; 0 0 1 0 0 0; 0 0 0 0 14 0]
  Left Motor : Subsystem  mask{vparams=p1_params.m}
      mask prompts: vparams "Vehicle parameters file"
      mask init:
      | % Load vehicle parameters file
      | evalc(strrep(vparams,'.m',''));
  Mux1 : Mux  Inputs=2
  Mux2 : Mux  Inputs=2
  Mux5 : Mux  Inputs=2
  Right Motor : Subsystem  mask{vparams=p1_params.m}
      mask prompts: vparams "Vehicle parameters file"
      mask init:
      | % Load vehicle parameters file
      | evalc(strrep(vparams,'.m',''));
  Sum1 : Sum  Inputs=++|  SaturateOnIntegerOverflow=on
  Angles : Outport
  Sensed Angles : Outport  Port=2
  Currents : Outport  Port=3
  wires:
  Demux2/2 -> Right Motor/3(Current Input)
  Demux2/1 -> Left Motor/3(Current Input)
  Current Input/1 -> Demux2/1
  Load Torques/1 -> Demux1/1
  Demux1/1 -> Left Motor/2(Load Torque)
  Demux1/2 -> Right Motor/2(Load Torque)
  Left Motor/1(Angle) -> Mux5/1
  Right Motor/1(Angle) -> Mux5/2
  Left Motor/2(Current Ouput) -> Mux1/1
  Right Motor/2(Current Ouput) -> Mux1/2
  Mux5/1 -> Angles/1, Sum1/1
  Mux1/1 -> Currents/1
  Direct Look-Up Table (n-D)/1 -> Demux3/1
  Fault/1 -> Direct Look-Up Table (n-D)/1
  Demux3/1 -> Left Motor/1(Fault)
  Demux3/3 -> Right Motor/1(Fault)
  Demux3/2 -> Mux2/1
  Demux3/4 -> Mux2/2
  Mux2/1 -> Sum1/2
  Sum1/1 -> Sensed Angles/1

== system VehicleSimulation/Vehicle Simulation/Driver/Handwheel System/HAL-9000/Double chirp/Chirp One ==
  note: freqSlope = deltaFreq/targetTime;
      | instantaneousFreq(t) = freqSlope*t + initialFreq;
      | intantaneousPhase(t) = integral(instFreq) = ...
      |       0.5*freqSlope*t^2 + initialFreq*t;
      | outputSignal(t) = sin(instantaneousPhase(t));
  Start Time : Inport
  Clock1 : Clock
      settings: DisableCoverage=on
  Gain : Gain  DisableCoverage=on  Gain=0.5  OutDataTypeStr=Inherit: Same as input  ParamDataTypeStr=Inherit: Same as input
  Output : Trigonometry
  Product : Product  DisableCoverage=on  Inputs=*/  SaturateOnIntegerOverflow=on  InputSameDT=on  OutDataTypeStr=Inherit: Same as first input
  Product1 : Product  DisableCoverage=on  SaturateOnIntegerOverflow=on  InputSameDT=on  OutDataTypeStr=Inherit: Same as first input
  Product2 : Product  DisableCoverage=on  SaturateOnIntegerOverflow=on  InputSameDT=on  OutDataTypeStr=Inherit: Same as first input
  Saturation : Saturate  UpperLimit=duration/2  LowerLimit=0
  Sum : Sum  DisableCoverage=on  Inputs=|++  SaturateOnIntegerOverflow=on  InputSameDT=on  OutDataTypeStr=Inherit: Same as first input
  Sum1 : Sum  DisableCoverage=on  Inputs=-+|  SaturateOnIntegerOverflow=on  InputSameDT=on  OutDataTypeStr=Inherit: Same as first input
  deltaFreq : Constant  DisableCoverage=on  Value=2*pi*(f2-f1)
  initialFreq : Constant  DisableCoverage=on  Value=2*pi*f1
  targetTime : Constant  DisableCoverage=on  Value=T
  Out2 : Outport
  wires:
  Sum1/1 -> Saturation/1
  Clock1/1 -> Sum1/2
  Start Time/1 -> Sum1/1
  deltaFreq/1 -> Product/1
  targetTime/1 -> Product/2
  Product/1 -> Gain/1
  Gain/1 -> Product1/2
  Product1/1 -> Sum/1
  initialFreq/1 -> Sum/2
  Sum/1 -> Product2/2
  Product2/1 -> Output/1
  Output/1 -> Out2/1
  Saturation/1 -> Product1/1, Product2/1

== system VehicleSimulation/Vehicle Simulation/Driver/Handwheel System/HAL-9000/Double chirp/Chirp Two ==
  note: freqSlope = deltaFreq/targetTime;
      | instantaneousFreq(t) = freqSlope*t + initialFreq;
      | intantaneousPhase(t) = integral(instFreq) = ...
      |       0.5*freqSlope*t^2 + initialFreq*t;
      | outputSignal(t) = sin(instantaneousPhase(t));
  Start Time : Inport
  Clock1 : Clock
      settings: DisableCoverage=on
  Gain : Gain  DisableCoverage=on  Gain=0.5  OutDataTypeStr=Inherit: Same as input  ParamDataTypeStr=Inherit: Same as input
  Output : Trigonometry
  Product : Product  DisableCoverage=on  Inputs=*/  SaturateOnIntegerOverflow=on  InputSameDT=on  OutDataTypeStr=Inherit: Same as first input
  Product1 : Product  DisableCoverage=on  SaturateOnIntegerOverflow=on  InputSameDT=on  OutDataTypeStr=Inherit: Same as first input
  Product2 : Product  DisableCoverage=on  SaturateOnIntegerOverflow=on  InputSameDT=on  OutDataTypeStr=Inherit: Same as first input
  Saturation : Saturate  UpperLimit=duration/2  LowerLimit=0
  Sum : Sum  DisableCoverage=on  Inputs=|++  SaturateOnIntegerOverflow=on  InputSameDT=on  OutDataTypeStr=Inherit: Same as first input
  Sum1 : Sum  DisableCoverage=on  Inputs=-+|  SaturateOnIntegerOverflow=on  InputSameDT=on  OutDataTypeStr=Inherit: Same as first input
  deltaFreq : Constant  DisableCoverage=on  Value=2*pi*(f2-f1)
  initialFreq : Constant  DisableCoverage=on  Value=2*pi*f1
  targetTime : Constant  DisableCoverage=on  Value=T
  Out2 : Outport
  wires:
  Sum1/1 -> Saturation/1
  Clock1/1 -> Sum1/2
  Start Time/1 -> Sum1/1
  deltaFreq/1 -> Product/1
  targetTime/1 -> Product/2
  Product/1 -> Gain/1
  Gain/1 -> Product1/2
  Product1/1 -> Sum/1
  initialFreq/1 -> Sum/2
  Sum/1 -> Product2/2
  Product2/1 -> Output/1
  Output/1 -> Out2/1
  Saturation/1 -> Product1/1, Product2/1

== system VehicleSimulation/Vehicle Simulation/Vehicle Model/Steering System Model/Electrical Components and Motors/Amplifiers/Left Amplifier ==
  Current Command : Inport
  Current Input : Outport
  wires:
  Current Command/1 -> Current Input/1

== system VehicleSimulation/Vehicle Simulation/Vehicle Model/Steering System Model/Electrical Components and Motors/Amplifiers/Right Amplifier ==
  Current Command1 : Inport
  Current Input : Outport
  wires:
  Current Command1/1 -> Current Input/1
